simulink model "comprehensive_model_with_rocks_trial"  (R2019a)
settings: Solver=FixedStepAuto  StartTime=0.0  StopTime=15  FixedStep=0.001  RelTol=1e-3
PreLoadFcn:
  | load('tumbleweed_constants.mat')
values from neighbouring files (symbols this model uses):
  Ar = 0.785398163397    [tumbleweed_constants.mat]
  CD = 0.8    [tumbleweed_constants.mat]
  d = 0.65    [tumbleweed_constants.mat]
  g = 9.81    [tumbleweed_constants.mat]
  Ixx = 1.29    [tumbleweed_constants.mat]
  Iyy = 1.29    [tumbleweed_constants.mat]
  Izz = 1.29    [tumbleweed_constants.mat]
  m = 1    [tumbleweed_constants.mat]
  maxr = 0.45    [tumbleweed_constants.mat]
  mf = 14    [tumbleweed_constants.mat]
  minr = 0.2    [tumbleweed_constants.mat]
  mu0 = 0.02    [tumbleweed_constants.mat]
  muk = 0.5    [tumbleweed_constants.mat]
  must = 0.8    [tumbleweed_constants.mat]
  R = cylR*ones(size(Theta,1),size(Theta,2))    [d3_animate.m]    (also in tumbleweed_constants.mat = 0.5)
  rest_coeff = 0.6    [tumbleweed_constants.mat]
  rho = 1.2    [tumbleweed_constants.mat]
  ts = 0.5    [tumbleweed_constants.mat]
  v_thres = 0.0001    [tumbleweed_constants.mat]
  vmax = 0.2    [tumbleweed_constants.mat]
  YY = 50    [tumbleweed_constants.mat]
libraries: simulink x2
(part 7 of 9)

== matlab function comprehensive_model_with_rocks_trial/bouncing_model1/onsurface_model/MATLAB Function9 ==
  data: t input; states0 output; roll_reset_flag output; states input; u input; r_RO input; rock_coll_flag input; rock_pardiffs input; jRp input; jR output; rest_coeff parameter; m parameter; mf parameter; Ixx parameter; d parameter; R parameter; must parameter; muk parameter; Iyy parameter; Izz parameter
function [states0, roll_reset_flag, jR] = rock_collision_state_set(t,states,u, r_RO, rock_coll_flag, rock_pardiffs, jRp, rest_coeff, m, mf, Ixx, d, R, must, muk, Iyy, Izz)
%u1 u2 u3 u4 u5 u6 S1 S2 S3
roll_reset_flag = 0;
O_w_T = [states(1);states(2);states(3)];
O_v_TO = [states(4);states(5);states(6)];
r_TO = [states(7);states(8);states(9)];
q = [states(10);states(11);states(12);states(13)];
q0 = q(1); q1 = q(2); q2 = q(3); q3 = q(4);

        fx = rock_pardiffs(1,1); 
        fy = rock_pardiffs(2,1);
        fz = rock_pardiffs(3,1);
        kO = [0;0;1];
        iO = [1;0;0];
        jO = [0;1;0];

        if(abs(fx)<=1e-20 && abs(fy) <= 1e-20)
            kR = kO;
            jR = jO;
            iR = iO;
            O_c_R = eye(3);
            R_c_O = eye(3);
            flag = 1;
        else
        kR = [fx;fy;fz]/norm([fx;fy;fz]);
        jR = cross(kO,kR)/norm(cross(kO,kR));
        flag = 1;
        if((jRp.')*(jR) < 0)
            jR = -jR;
            flag = 2;
        end
        iR = cross(jR,kR);
        R_c_O = [iR'*iO, iR'*jO, iR'*kO; jR'*iO, jR'*jO, jR'*kO; kR'*iO, kR'*jO, kR'*kO];
        O_c_R = transpose(R_c_O);
        end
O_v_TOr = R_c_O*O_v_TO;       

if rock_coll_flag == 0
    jR = [0;1;0];
end
        
if mod(t,0.001) == 0 && rock_coll_flag == 1
 %%collision response
     
        T_c_O = [q0^2 + q1^2 - q2^2 - q3^2, 2*(q1*q2 + q0*q3), 2*(q1*q3 - q0*q2);...
        2*(q1*q2 - q0*q3), q0^2 - q1^2 + q2^2 - q3^2, 2*(q2*q3 + q0*q1);...
        2*(q1*q3 + q0*q2), 2*(q2*q3 - q0*q1), q0^2 - q1^2 - q2^2 + q3^2];
        O_c_T = T_c_O.';
       
        
        
        T_c_R = T_c_O*O_c_R;
        R_c_T = T_c_R.';
        
        l1 = u(1); l2 = u(2); l3 = u(3); l4 = u(4); l5 = u(5); l6 = u(6);
        L33 = Ixx + m*(l3^2 + l4^2 + l5^2 + l6^2);
        L11 = Iyy + m*(l1^2 + l2^2 + l5^2 + l6^2);
        L22 = Izz + m*(l3^2 + l4^2 + l1^2 + l2^2);
        L = R_c_T*[L33,0,0;0,L11,0;0,0,L22]*T_c_R;
        L11 = L(2,2);
        L22 = L(3,3);
        L33 = L(1,1);
        mT = mf +6*m;

        w = R_c_T*(O_w_T);
        v = R_c_O*O_v_TO;

        u3 = w(1,1);
        u2 = w(3,1);
        u1 = w(2,1);

        u6 = v(1,1);
        u5 = v(3,1);
        u4 = v(2,1);


        u5_n = -rest_coeff*u5;  

        roll_reset_flag = 1;
        r_TO = r_RO + R*kR;
        
        u2_n = u2;
        u3_n = (L33*u3 - mT*R*u4)/(mT*R^2 + L33);
        u4_n = -R*u3_n;
        u1_n = (L11*u1 + mT*R*u6)/(mT*R^2 + L11);
        u6_n = R*u1_n;
        S1 = mT*(u4_n - u4);
        S2 = mT*(u5_n - u5);
        S3 = mT*(u6_n - u6);

        if ~(sqrt(S1^2 + S3^2) < must*norm(S2))
            alpha = u4 + R*u3;
            gamma = u6 - R*u1;
            k1 = 1/mT + R^2/L11;
            k3 = 1/mT + R^2/L33;
            
            if abs(alpha) > 0
                S1 = S1solve(S2, muk,alpha, gamma, k1, k3); 
                S3 = gamma*S1/(alpha + (k3 - k1)*S1);
                u1_n = u1 - R*S3/L11;
                u3_n = u3 + R*S1/L33;
                u4_n = u4 + S1/mT;
                u6_n = u6 + S3/mT;
            else 
                S3 = S1solve(S2, muk, gamma, alpha, k3, k1);
                S1 = alpha*S3/(gamma + (k1 - k3)*S3);
                u1_n = u1 - R*S3/L11;
                u3_n = u3 + R*S1/L33;
                u4_n = u4 + S1/mT;
                u6_n = u6 + S3/mT;
            end
            
        end

        O_w_T = T_c_R*[u3_n;u1_n;u2_n];
        O_v_TO = O_c_R*[u6_n; u4_n; u5_n];
end

states0 = [O_w_T;O_v_TO;r_TO;q];

end
